simulink model "sim1"  (R2015b)
settings: Solver=VariableStepAuto  StartTime=0.0  StopTime=10.0  RelTol=1e-3
settings Model: Creator=29118  LastModifiedBy=朱明菲

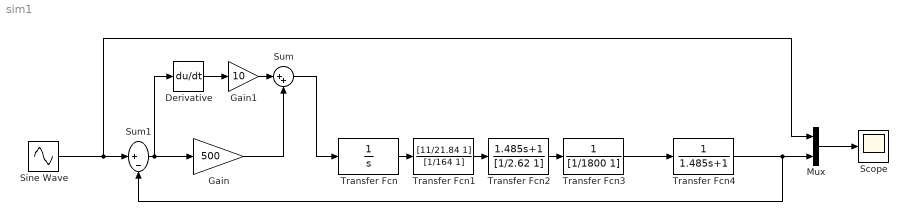
== system sim1 ==
  Derivative : Derivative
  Gain : Gain  Gain=500
  Gain1 : Gain  Gain=10
  Mux : Mux  Inputs=2
  Scope : Scope
  Sine Wave : Sin  SampleTime=0
  Sum : Sum  Inputs=|++
  Sum1 : Sum  Inputs=|+-
  Transfer Fcn : TransferFcn  Denominator=[1 0]
  Transfer Fcn1 : TransferFcn  Numerator=[11/21.84 1]  Denominator=[1/164 1]
  Transfer Fcn2 : TransferFcn  Numerator=[1.485 1]  Denominator=[1/2.62 1]
  Transfer Fcn3 : TransferFcn  Denominator=[1/1800 1]
  Transfer Fcn4 : TransferFcn  Denominator=[1.485 1 ]
  wires:
  Mux/1 -> Scope/1
  Transfer Fcn3/1 -> Transfer Fcn4/1
  Transfer Fcn/1 -> Transfer Fcn1/1
  Transfer Fcn1/1 -> Transfer Fcn2/1
  Transfer Fcn2/1 -> Transfer Fcn3/1
  Sine Wave/1 -> Mux/1, Sum1/1
  Gain/1 -> Sum/2
  Sum/1 -> Transfer Fcn/1
  Derivative/1 -> Gain1/1
  Gain1/1 -> Sum/1
  Transfer Fcn4/1 -> Sum1/2, Mux/2
  Sum1/1 -> Gain/1, Derivative/1
